simulink model "Einfache_Zustandsrueckfuehrung_linear"  (R2021b)
settings: Solver=FixedStepAuto  StartTime=0.0  StopTime=10.0  FixedStep=1/1e4  RelTol=1e-3
undefined symbols (not defined in the file): A, B, C, k, start_deg, V_m, x_c
settings Model: Creator=basti  LastModifiedBy=basti

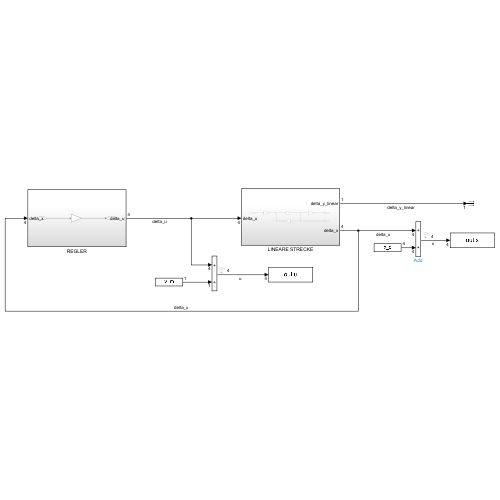
[thumbnail: Simulink's stored preview of the top-level diagram]
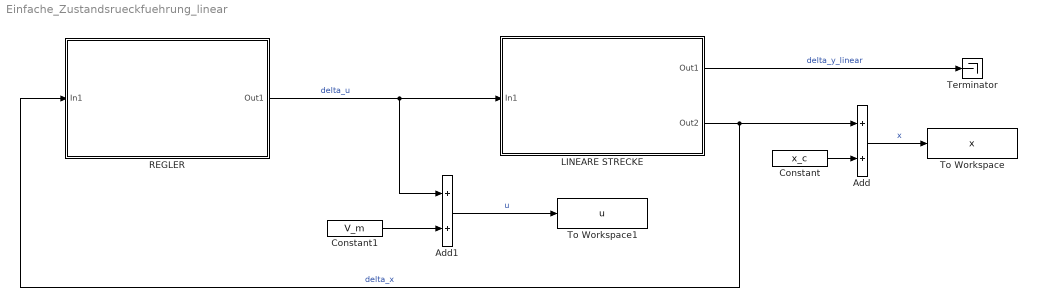
== system Einfache_Zustandsrueckfuehrung_linear ==
  Add : Sum
  Add1 : Sum
  Constant : Constant  Value=x_c
  Constant1 : Constant  Value=V_m
  LINEARE STRECKE : Subsystem
  REGLER : Subsystem
  Terminator : Terminator
  To Workspace : ToWorkspace  VariableName=x  SaveFormat=Timeseries  SampleTime=-1
  To Workspace1 : ToWorkspace  VariableName=u  SaveFormat=Timeseries  SampleTime=-1
  wires:
  REGLER/1(Out1) -> LINEARE STRECKE/1(In1), Add1/1  "delta_u"
  LINEARE STRECKE/1(Out1) -> Terminator/1  "delta_y_linear"
  LINEARE STRECKE/2(Out2) -> REGLER/1(In1), Add/1  "delta_x"
  Constant/1 -> Add/2
  Add/1 -> To Workspace/1  "x"
  Constant1/1 -> Add1/2
  Add1/1 -> To Workspace1/1  "u"

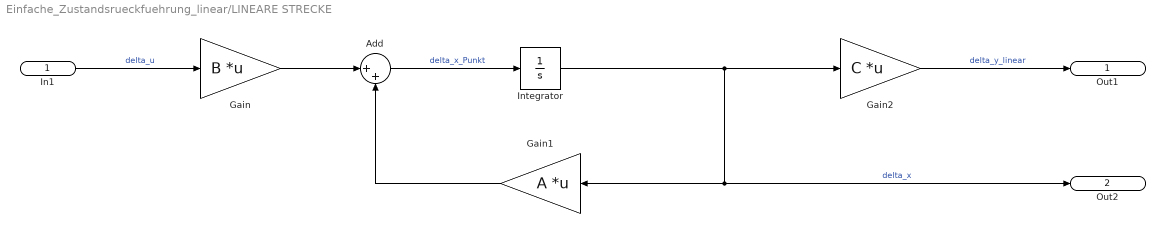
== system Einfache_Zustandsrueckfuehrung_linear/LINEARE STRECKE ==
  In1 : Inport
  Add : Sum  Inputs=|++
  Gain : Gain  Gain=B  Multiplication=Matrix(K*u) (u vector)
  Gain1 : Gain  Gain=A  Multiplication=Matrix(K*u) (u vector)
  Gain2 : Gain  Gain=C  Multiplication=Matrix(K*u) (u vector)
  Integrator : Integrator  InitialCondition=[(start_deg*pi/180); 0; 0; 0]
  Out1 : Outport
  Out2 : Outport  Port=2
  wires:
  Gain/1 -> Add/1
  Integrator/1 -> Gain2/1, Gain1/1, Out2/1  "delta_x"
  Add/1 -> Integrator/1  "delta_x_Punkt"
  Gain1/1 -> Add/2
  In1/1 -> Gain/1  "delta_u"
  Gain2/1 -> Out1/1  "delta_y_linear"

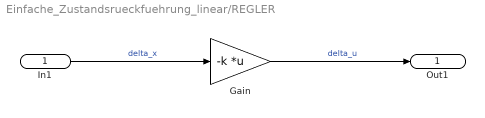
== system Einfache_Zustandsrueckfuehrung_linear/REGLER ==
  In1 : Inport
  Gain : Gain  Gain=-k  Multiplication=Matrix(K*u) (u vector)
  Out1 : Outport
  wires:
  In1/1 -> Gain/1  "delta_x"
  Gain/1 -> Out1/1  "delta_u"
